simulink model "fangzhen2"  (R2014a)
settings: Solver=ode45  StartTime=0.0  StopTime=5  RelTol=1e-3
settings Model: Creator=HZQ  LastModifiedBy=pengpeng

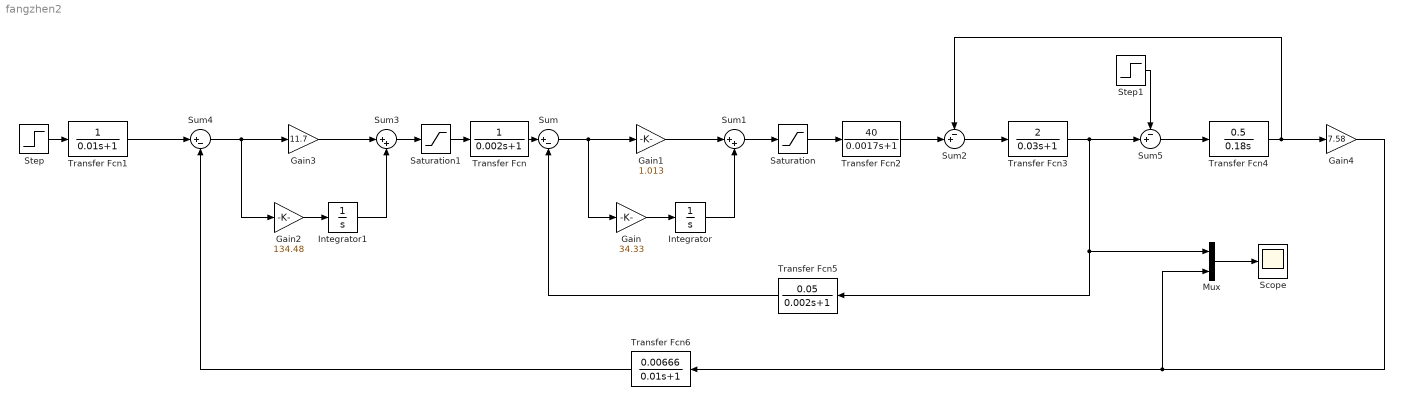
== system fangzhen2 ==
  Gain : Gain  Gain=34.33
  Gain1 : Gain  Gain=1.013
  Gain2 : Gain  Gain=134.48
  Gain3 : Gain  Gain=11.7
  Gain4 : Gain  Gain=7.58
  Integrator : Integrator
  Integrator1 : Integrator  LimitOutput=on  UpperSaturationLimit=10  LowerSaturationLimit=-10
  Mux : Mux  Inputs=2
  Saturation : Saturate  UpperLimit=10  LowerLimit=-10
  Saturation1 : Saturate  UpperLimit=10  LowerLimit=-10
  Scope : Scope
      settings: TimeRange=2
  Step : Step  Before=10  After=10  SampleTime=0
  Step1 : Step  Before=10  After=0  SampleTime=0
  Sum : Sum  Inputs=|+-
  Sum1 : Sum  Inputs=|++
  Sum2 : Sum  Inputs=-+|
  Sum3 : Sum  Inputs=|++
  Sum4 : Sum  Inputs=|+-
  Sum5 : Sum  Inputs=-+|
  Transfer Fcn : TransferFcn  Denominator=[0.002 1]
  Transfer Fcn1 : TransferFcn  Denominator=[0.01 1]
  Transfer Fcn2 : TransferFcn  Numerator=[40]  Denominator=[0.0017 1]
  Transfer Fcn3 : TransferFcn  Numerator=[2]  Denominator=[0.03 1]
  Transfer Fcn4 : TransferFcn  Numerator=[0.5]  Denominator=[0.18 0]
  Transfer Fcn5 : TransferFcn  Numerator=[0.05]  Denominator=[0.002 1]
  Transfer Fcn6 : TransferFcn  Numerator=[0.00666]  Denominator=[0.01 1]
  wires:
  Transfer Fcn/1 -> Sum/1
  Sum/1 -> Gain1/1, Gain/1
  Gain/1 -> Integrator/1
  Gain1/1 -> Sum1/1
  Integrator/1 -> Sum1/2
  Transfer Fcn2/1 -> Sum2/2
  Sum2/1 -> Transfer Fcn3/1
  Sum1/1 -> Saturation/1
  Saturation/1 -> Transfer Fcn2/1
  Transfer Fcn3/1 -> Sum5/2, Mux/1, Transfer Fcn5/1
  Transfer Fcn4/1 -> Gain4/1, Sum2/1
  Transfer Fcn5/1 -> Sum/2
  Gain2/1 -> Integrator1/1
  Gain3/1 -> Sum3/1
  Integrator1/1 -> Sum3/2
  Step/1 -> Transfer Fcn1/1
  Transfer Fcn1/1 -> Sum4/1
  Transfer Fcn6/1 -> Sum4/2
  Sum4/1 -> Gain2/1, Gain3/1
  Sum5/1 -> Transfer Fcn4/1
  Step1/1 -> Sum5/1
  Gain4/1 -> Mux/2, Transfer Fcn6/1
  Saturation1/1 -> Transfer Fcn/1
  Sum3/1 -> Saturation1/1
  Mux/1 -> Scope/1
